simulink subsystem "Subsystem_Plant_BAv01"  (R2022b)
settings: Solver=VariableStepAuto  StartTime=0.0  StopTime=10.0  RelTol=1e-3
undefined symbols (not defined in the file): driver, getPhysicalConstants, param, route
settings Model: Creator=giaco  LastModifiedBy=giaco

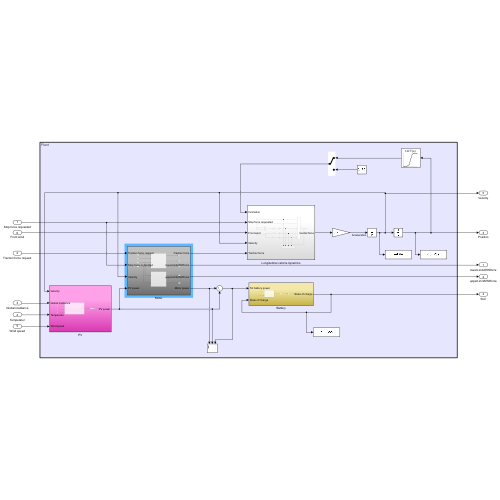
[thumbnail: Simulink's stored preview of the top-level diagram]
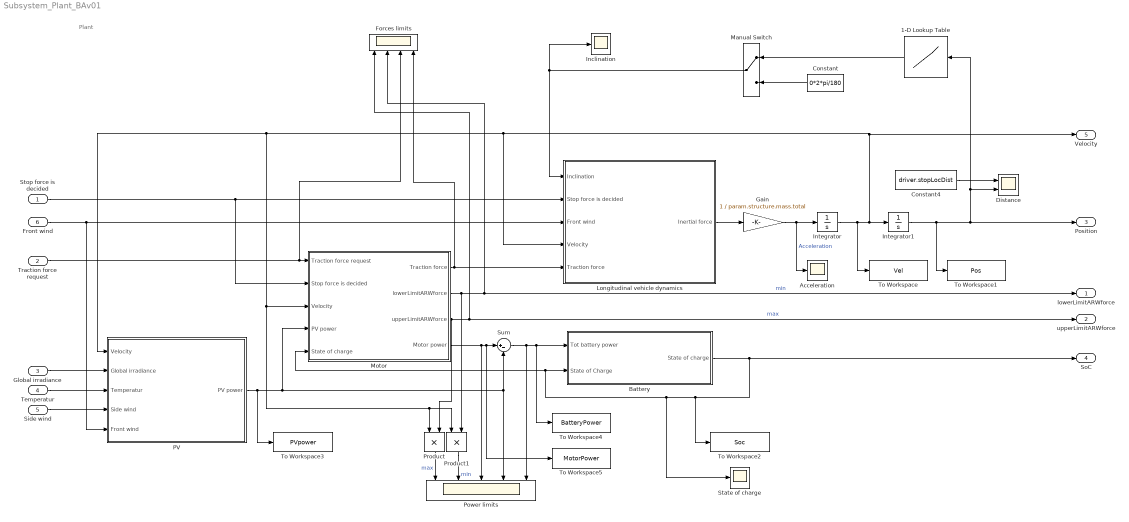
== system Subsystem_Plant_BAv01 ==
  note: Plant
  Stop force is decided : Inport
  Traction force request : Inport  Port=2
  Global irradiance : Inport  Port=3
  Temperatur : Inport  Port=4
  Side wind : Inport  Port=5
  Front wind : Inport  Port=6
  1-D Lookup Table : Lookup_n-D  NumberOfTableDimensions=1  BreakpointsForDimension1=route.dist(1:end-1)  Table=route.inclSmooth  InternalRulePriority=Speed  RndMeth=Simplest
  Acceleration : Scope
  Battery : Subsystem
  Constant : Constant  Value=0*2*pi/180
  Constant4 : Constant  Value=driver.stopLocDist
  Distance : Scope  NumInputPorts=2
  Forces limits : Scope  NumInputPorts=4
  Gain : Gain  Gain=1 / param.structure.mass.total
  Inclination : Scope
  Integrator : Integrator
  Integrator1 : Integrator
  Longitudinal vehicle dynamics : Subsystem
  Manual Switch : ManualSwitch
  Motor : Subsystem
  PV : Subsystem
  Power limits : Scope  NumInputPorts=5
  Product : Product
  Product1 : Product
  State of charge : Scope
  Sum : Sum  Inputs=|+-
  To Workspace : ToWorkspace  VariableName=Vel  SaveFormat=Timeseries  SampleTime=-1
  To Workspace1 : ToWorkspace  VariableName=Pos  SaveFormat=Timeseries  SampleTime=-1
  To Workspace2 : ToWorkspace  VariableName=Soc  SaveFormat=Timeseries  SampleTime=-1
  To Workspace3 : ToWorkspace  VariableName=PVpower  SaveFormat=Timeseries  SampleTime=-1
  To Workspace4 : ToWorkspace  VariableName=BatteryPower  SaveFormat=Timeseries  SampleTime=-1
  To Workspace5 : ToWorkspace  VariableName=MotorPower  SaveFormat=Timeseries  SampleTime=-1
  lowerLimitARWforce : Outport
  upperLimitARWforce : Outport  Port=2
  Position : Outport  Port=3
  SoC : Outport  Port=4
  Velocity : Outport  Port=5
  wires:
  Integrator/1 -> To Workspace/1, Velocity/1, Longitudinal vehicle dynamics/4(Velocity), PV/1(Velocity), Product/1, Product1/1, Motor/3(Velocity), Integrator1/1
  Battery/1(State of charge) -> SoC/1, To Workspace2/1, Motor/5(State of charge), Battery/2(State of Charge), State of charge/1
  Longitudinal vehicle dynamics/1(Inertial force) -> Gain/1
  Manual Switch/1 -> Longitudinal vehicle dynamics/1(Inclination), Inclination/1
  Traction force request/1 -> Motor/1(Traction force request), Forces limits/3
  Gain/1 -> Integrator/1, Acceleration/1  "Acceleration"
  Sum/1 -> Power limits/5, Battery/1(Tot battery power), To Workspace4/1
  Integrator1/1 -> To Workspace1/1, Distance/2, 1-D Lookup Table/1, Position/1
  PV/1(PV power) -> Power limits/4, Sum/2, Motor/4(PV power), To Workspace3/1
  1-D Lookup Table/1 -> Manual Switch/1
  Motor/4(Motor power) -> Power limits/3, Sum/1, To Workspace5/1
  Stop force is decided/1 -> Motor/2(Stop force is decided), Longitudinal vehicle dynamics/2(Stop force is decided)
  Constant/1 -> Manual Switch/2
  Motor/1(Traction force) -> Longitudinal vehicle dynamics/5(Traction force), Forces limits/4
  Global irradiance/1 -> PV/2(Global irradiance)
  Temperatur/1 -> PV/3(Temperatur)
  Side wind/1 -> PV/4(Side wind)
  Front wind/1 -> PV/5(Front wind), Longitudinal vehicle dynamics/3(Front wind)
  Product/1 -> Power limits/1  "max"
  Product1/1 -> Power limits/2  "min"
  Motor/3(upperLimitARWforce) -> Product/2, upperLimitARWforce/1, Forces limits/1  "max"
  Motor/2(lowerLimitARWforce) -> Product1/2, Forces limits/2, lowerLimitARWforce/1  "min"
  Constant4/1 -> Distance/1

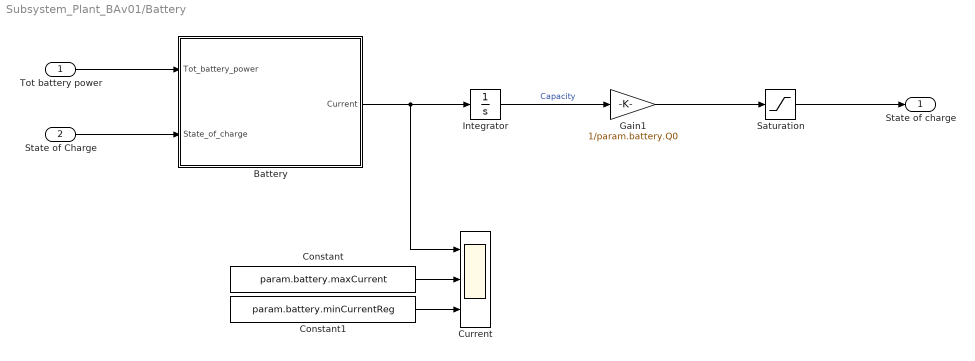
== system Subsystem_Plant_BAv01/Battery ==
  Tot battery power : Inport
  State of Charge : Inport  Port=2
  Battery : MATLAB Function  TreatAsAtomicUnit=on
  Constant : Constant  Value=param.battery.maxCurrent
  Constant1 : Constant  Value=param.battery.minCurrentReg
  Current : Scope  NumInputPorts=3
  Gain1 : Gain  Gain=1/param.battery.Q0
  Integrator : Integrator  InitialCondition=param.battery.Q0 / 100 * 100
  Saturation : Saturate  UpperLimit=1  LowerLimit=-Inf
  State of charge : Outport
  wires:
  Constant1/1 -> Current/3
  Constant/1 -> Current/2
  State of Charge/1 -> Battery/2(State_of_charge)
  Battery/1(Current) -> Integrator/1, Current/1
  Integrator/1 -> Gain1/1  "Capacity"
  Gain1/1 -> Saturation/1
  Tot battery power/1 -> Battery/1(Tot_battery_power)
  Saturation/1 -> State of charge/1

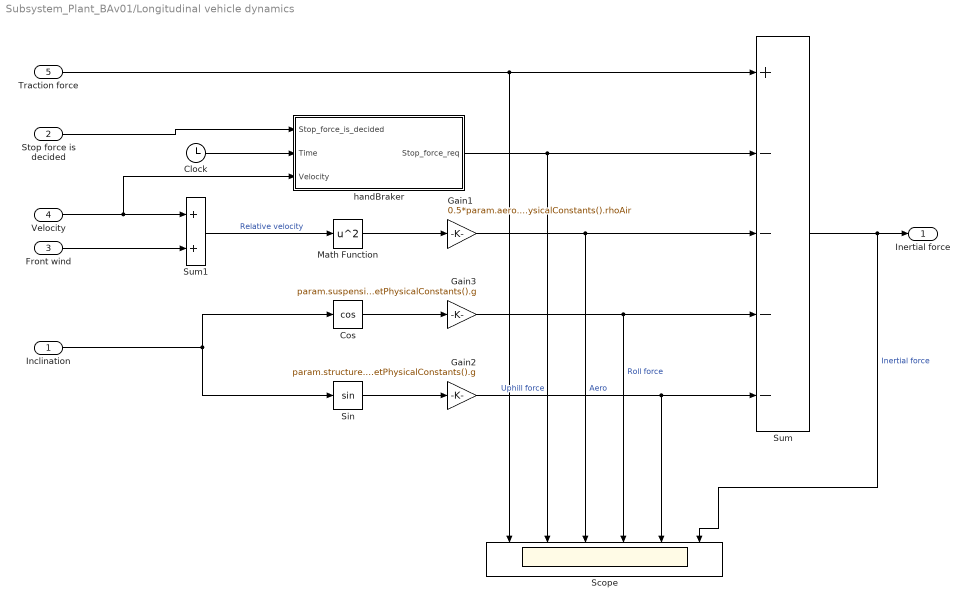
== system Subsystem_Plant_BAv01/Longitudinal vehicle dynamics ==
  Inclination : Inport
  Stop force is decided : Inport  Port=2
  Front wind : Inport  Port=3
  Velocity : Inport  Port=4
  Traction force : Inport  Port=5
  Clock : Clock
  Cos : Trigonometry  Operator=cos
  Gain1 : Gain  Gain=0.5*param.aero.AfCd*getPhysicalConstants().rhoAir
  Gain2 : Gain  Gain=param.structure.mass.total*getPhysicalConstants().g
  Gain3 : Gain  Gain=param.suspension.cR*param.structure.mass.total*getPhysicalConstants().g
  Math Function : Math  Operator=square
  Scope : Scope  NumInputPorts=6
  Sin : Trigonometry
  Sum : Sum  Inputs=+----
  Sum1 : Sum
  handBraker : MATLAB Function  TreatAsAtomicUnit=on
  Inertial force : Outport
  wires:
  Clock/1 -> handBraker/2(Time)
  Stop force is decided/1 -> handBraker/1(Stop_force_is_decided)
  Traction force/1 -> Sum/1, Scope/1
  Gain1/1 -> Sum/3, Scope/3  "Aero"
  Gain3/1 -> Sum/4, Scope/4  "Roll force"
  Cos/1 -> Gain3/1
  Math Function/1 -> Gain1/1
  Inclination/1 -> Cos/1, Sin/1
  Sin/1 -> Gain2/1
  Gain2/1 -> Sum/5, Scope/5  "Uphill force"
  Velocity/1 -> Sum1/1, handBraker/3(Velocity)
  Sum/1 -> Inertial force/1, Scope/6  "Inertial force"
  handBraker/1(Stop_force_req) -> Sum/2, Scope/2
  Front wind/1 -> Sum1/2
  Sum1/1 -> Math Function/1  "Relative velocity"

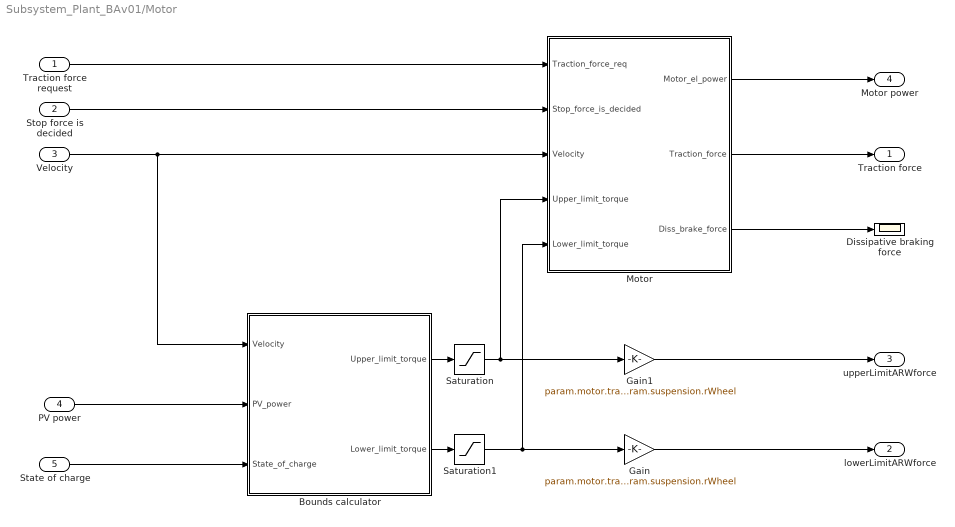
== system Subsystem_Plant_BAv01/Motor ==
  Traction force request : Inport
  Stop force is decided : Inport  Port=2
  Velocity : Inport  Port=3
  PV power : Inport  Port=4
  State of charge : Inport  Port=5
  Bounds calculator : MATLAB Function  TreatAsAtomicUnit=on
  Dissipative braking force : Scope
  Gain : Gain  Gain=param.motor.transmissionRatio / param.suspension.rWheel
  Gain1 : Gain  Gain=param.motor.transmissionRatio / param.suspension.rWheel
  Motor : MATLAB Function  TreatAsAtomicUnit=on
  Saturation : Saturate  UpperLimit=Inf  LowerLimit=0
  Saturation1 : Saturate  UpperLimit=0  LowerLimit=-Inf
  Traction force : Outport
  lowerLimitARWforce : Outport  Port=2
  upperLimitARWforce : Outport  Port=3
  Motor power : Outport  Port=4
  wires:
  Saturation1/1 -> Gain/1, Motor/5(Lower_limit_torque)
  Saturation/1 -> Gain1/1, Motor/4(Upper_limit_torque)
  Bounds calculator/1(Upper_limit_torque) -> Saturation/1
  Bounds calculator/2(Lower_limit_torque) -> Saturation1/1
  State of charge/1 -> Bounds calculator/3(State_of_charge)
  Traction force request/1 -> Motor/1(Traction_force_req)
  Velocity/1 -> Motor/3(Velocity), Bounds calculator/1(Velocity)
  Motor/1(Motor_el_power) -> Motor power/1
  Motor/2(Traction_force) -> Traction force/1
  Motor/3(Diss_brake_force) -> Dissipative braking force/1
  PV power/1 -> Bounds calculator/2(PV_power)
  Stop force is decided/1 -> Motor/2(Stop_force_is_decided)
  Gain1/1 -> upperLimitARWforce/1
  Gain/1 -> lowerLimitARWforce/1

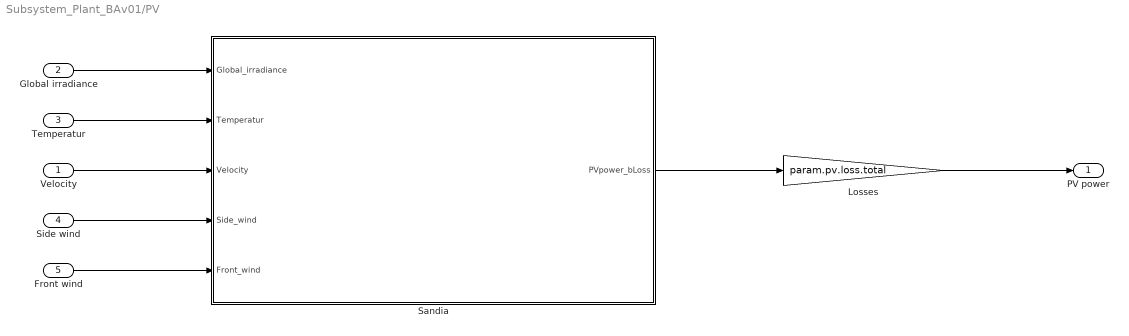
== system Subsystem_Plant_BAv01/PV ==
  Velocity : Inport
  Global irradiance : Inport  Port=2
  Temperatur : Inport  Port=3
  Side wind : Inport  Port=4
  Front wind : Inport  Port=5
  Losses : Gain  Gain=param.pv.loss.total
  Sandia : MATLAB Function  TreatAsAtomicUnit=on
  PV power : Outport
  wires:
  Front wind/1 -> Sandia/5(Front_wind)
  Global irradiance/1 -> Sandia/1(Global_irradiance)
  Temperatur/1 -> Sandia/2(Temperatur)
  Sandia/1(PVpower_bLoss) -> Losses/1
  Losses/1 -> PV power/1
  Velocity/1 -> Sandia/3(Velocity)
  Side wind/1 -> Sandia/4(Side_wind)

== matlab function Subsystem_Plant_BAv01/PV/Sandia ==
  data: Global_irradiance input; Temperatur input; Velocity input; PVpower_bLoss output; Side_wind input; Front_wind input; param parameter
function PVpower_bLoss = fcn(Global_irradiance, Temperatur, Velocity, Side_wind, Front_wind, param)

type = "glass-cell-polymer";
mounting = "open rack";

relVelocity = Velocity + Front_wind;
effVelocity = sqrt(relVelocity^2 + Side_wind^2);

tempCell = cellTemperatureSandia(Global_irradiance, Temperatur, effVelocity, type, mounting);

PVpower_bLoss = param.pv.area * Global_irradiance * param.pv.eff * (1 + param.pv.powerCoeff * (tempCell - param.pv.tempSTC));

== matlab function Subsystem_Plant_BAv01/Battery/Battery ==
  data: Tot_battery_power input; State_of_charge input; Current output; param parameter
function Current = fcn(Tot_battery_power, State_of_charge, param)

%conversion to single battery power
Battery_power = Tot_battery_power ./ param.battery.totNum;

%OC parameters
Uoc = param.battery.k2 .* State_of_charge + param.battery.k1;
Ri = param.battery.k4 .* State_of_charge + param.battery.k3;

%solution of quadratic equation
Current_befEff = (Uoc - sqrt(Uoc^2 - 4*Battery_power*Ri)) / (2*Ri);

%Coulomb efficiency
Current = -1 * param.battery.effCoul .* Current_befEff;

== matlab function Subsystem_Plant_BAv01/Longitudinal vehicle dynamics/handBraker ==
  data: Stop_force_is_decided input; Time input; Velocity input; Stop_force_req output
function Stop_force_req = handBraker(Stop_force_is_decided, Time, Velocity)

Stop_force_req = 0;

if Stop_force_is_decided || (Velocity < 0 && Time > 10)
    Stop_force_req = 1000 * sign(Velocity);
end % if

== matlab function Subsystem_Plant_BAv01/Motor/Bounds calculator ==
  data: Velocity input; PV_power input; State_of_charge input; param parameter; Upper_limit_torque output; Lower_limit_torque output
function [Upper_limit_torque, Lower_limit_torque] = boundsCalculator(Velocity, PV_power, State_of_charge, param)

%%  Conversion battery limits
minElPowerMotBat = param.battery.lowerBoundPower * param.battery.totNum + PV_power;
minMechPowerMotBat = elPower2mechPower_Willans(minElPowerMotBat, param);

maxElPowerMotBat = param.battery.upperBoundPower * param.battery.totNum + PV_power;
maxMechPowerMotBat = elPower2mechPower_Willans(maxElPowerMotBat, param);

%state of charge relation
SoCwendePunkt = 0.20; %-
if State_of_charge < SoCwendePunkt
    maxPowerSoC = maxMechPowerMotBat / SoCwendePunkt * State_of_charge;
else
    maxPowerSoC = maxMechPowerMotBat;
end % if

%% Torque and rotational speed
omegaMot = Velocity * param.motor.transmissionRatio/param.suspension.rWheel;

%% Lower limit
Lower_limit_torque = max(param.motor.minTorque, param.motor.minPower / max(omegaMot, 1e-8)); %lower limit power motor
Lower_limit_torque = max(Lower_limit_torque, minMechPowerMotBat / max(omegaMot, 1e-8)); %lower limit power battery

%% Upper limit
Upper_limit_torque = min(param.motor.maxTorque, param.motor.maxPower / max(omegaMot, 1e-8)); %upper limit power motor
Upper_limit_torque = min(Upper_limit_torque, maxMechPowerMotBat / max(omegaMot, 1e-8)); %upper limit power battery
Upper_limit_torque = min(Upper_limit_torque, maxPowerSoC / max(omegaMot, 1e-8)); %upper limit state of charge

%safety bounds
% if Upper_limit_torque <= 0
%     Upper_limit_torque = 0;
% 
% elseif Lower_limit_torque >= 0
%     Lower_limit_torque = 0;
% end % if

% if Upper_limit_torque < Lower_limit_torque
%     Upper_limit_torque = Lower_limit_torque;
% 
% elseif Lower_limit_torque > Upper_limit_torque
%     Lower_limit_torque = Upper_limit_torque;
% end % if
end % fct

== matlab function Subsystem_Plant_BAv01/Motor/Motor ==
  data: Traction_force_req input; Stop_force_is_decided input; Velocity input; Upper_limit_torque input; Lower_limit_torque input; param parameter; Motor_el_power output; Traction_force output; Diss_brake_force output
function [Motor_el_power, Traction_force, Diss_brake_force] = Motor(Traction_force_req, Stop_force_is_decided, Velocity, Upper_limit_torque, Lower_limit_torque, param)

Diss_brake_force = 0;

%% Standing condition
if Stop_force_is_decided
    Traction_force = 0;
    Motor_el_power = 0;

else
%% Conversions
    tractionTorqueReq = Traction_force_req * param.suspension.rWheel/param.motor.transmissionRatio;
    omegaMot = Velocity * param.motor.transmissionRatio/param.suspension.rWheel;

%% Limits
    tractionTorque = tractionTorqueReq;
    tractionTorque = min(tractionTorque, Upper_limit_torque); %upper limit
    tractionTorque = max(tractionTorque, Lower_limit_torque); %lower limit
    
%% Electric motor power
    mechPower = omegaMot * tractionTorque;
    Motor_el_power = mechPower2elPower_Willans(mechPower, param);

%% Traction force
    Traction_force = tractionTorque * param.motor.transmissionRatio / param.suspension.rWheel;

    %additional dissipative braking force
    deltaBrake = Traction_force_req - Traction_force;
    if deltaBrake < 0
        Diss_brake_force = deltaBrake;
        Traction_force = Traction_force + Diss_brake_force;
    end % if
end % if
end % fct
